simulink model "compare_plant_SIMO"  (R2022b)
settings: Solver=VariableStepAuto  StartTime=0.0  StopTime=100  RelTol=1e-3
values from neighbouring files (symbols this model uses):
  airspeed_trim = 13.8507137299    [airspeed_trim.mat]
  alt_trim = 556.973205566    [alt_trim.mat]
  elevator_trim = 0    [elevator_trim.mat]
  throttle_trim = 0.234714001417    [throttle_trim.mat]
undefined symbols (not defined in the file or in its folder): sigbuilder_block
libraries: simulink_extras x3, dspsrcs4 x1, cstblocks x1

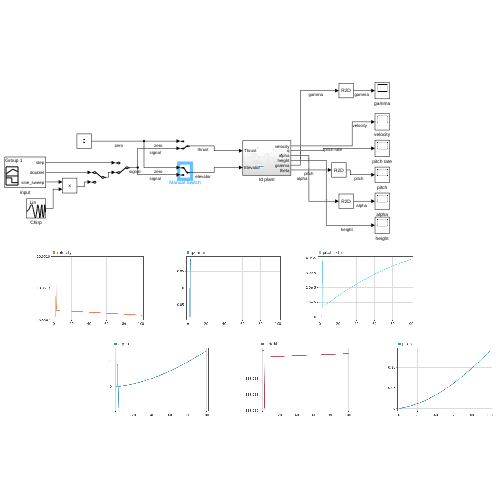
[thumbnail: Simulink's stored preview of the top-level diagram]
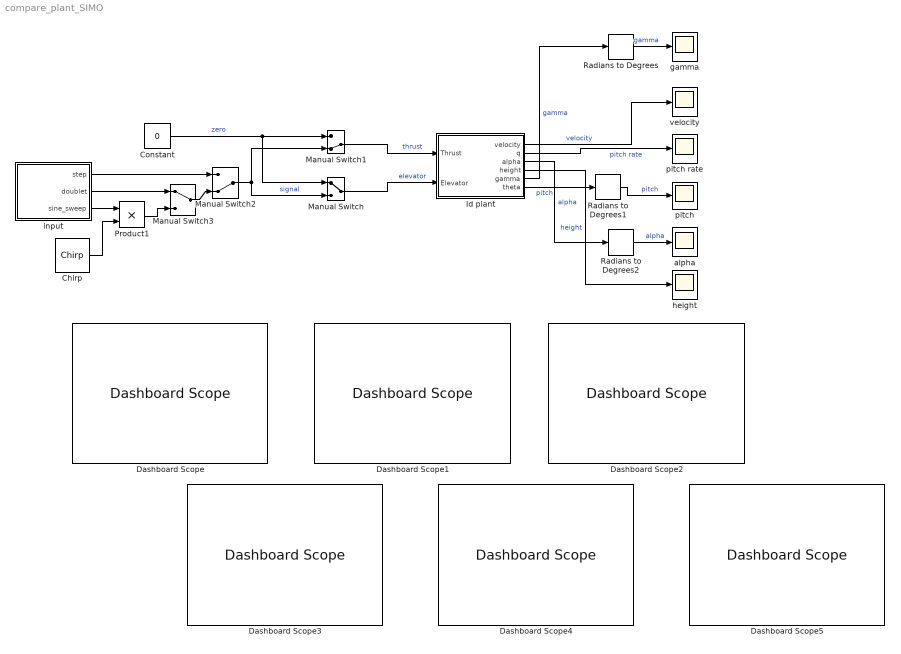
== system compare_plant_SIMO ==
  Chirp : dspsrcs4/Chirp  sweep=Linear  mode=Unidirectional  f0=0  f1=5  t1=20  Tsweep=20  phase=0  Ts=0.02  spf=1  datatype=Double  OutputFrames=off
  Constant : Constant  Value=0
  Dashboard Scope{,1..5} (6 alike) : DashboardScope
  Id plant : Subsystem
  Manual Switch : ManualSwitch
  Manual Switch1 : ManualSwitch  CurrentSetting=0
  Manual Switch2 : ManualSwitch  CurrentSetting=0
  Manual Switch3 : ManualSwitch
  Product1 : Product
  Radians to Degrees : simulink_extras/Transformations/Radians to Degrees
  Radians to Degrees1 : simulink_extras/Transformations/Radians to Degrees
  Radians to Degrees2 : simulink_extras/Transformations/Radians to Degrees
  alpha : Scope
  gamma : Scope
  height : Scope
  input : Subsystem  Tag=STV Subsys  LoadFcn=sigbuilder_block('load');  StartFcn=sigbuilder_block('start');  StopFcn=sigbuilder_block('stop');  ClipboardFcn=sigbuilder_block('clipboard');  mask(Sigbuilder block){tuvar=[0:10]}
      mask help: Simulink:masks:SigbuilderBlock_MD
      mask init:
      | if ~strcmp(get_param(bdroot(gcbh),'SimulationStatus'),'stopped') tuvar = sigbuilder_block('maskInit'); end
  pitch : Scope
  pitch rate : Scope
  velocity : Scope
  wires:
  Manual Switch1/1 -> Id plant/1(Thrust)  "thrust"
  Manual Switch/1 -> Id plant/2("Elevator ")  "elevator"
  Id plant/1(velocity) -> velocity/1  "velocity"
  Id plant/5(gamma) -> Radians to Degrees/1  "gamma"
  Id plant/2(q) -> pitch rate/1  "pitch rate"
  Id plant/3(alpha) -> Radians to Degrees2/1  "alpha"
  Id plant/4(height) -> height/1  "height"
  Product1/1 -> Manual Switch3/2
  Manual Switch2/1 -> Manual Switch/2, Manual Switch1/2  "signal"
  input/1(step) -> Manual Switch2/1
  Constant/1 -> Manual Switch/1, Manual Switch1/1  "zero"
  input/3(sine_sweep) -> Product1/1
  Chirp/1 -> Product1/2
  Id plant/6(theta) -> Radians to Degrees1/1  "pitch"
  Manual Switch3/1 -> Manual Switch2/2
  input/2(doublet) -> Manual Switch3/1
  Radians to Degrees/1 -> gamma/1  "gamma"
  Radians to Degrees1/1 -> pitch/1  "pitch"
  Radians to Degrees2/1 -> alpha/1  "alpha"

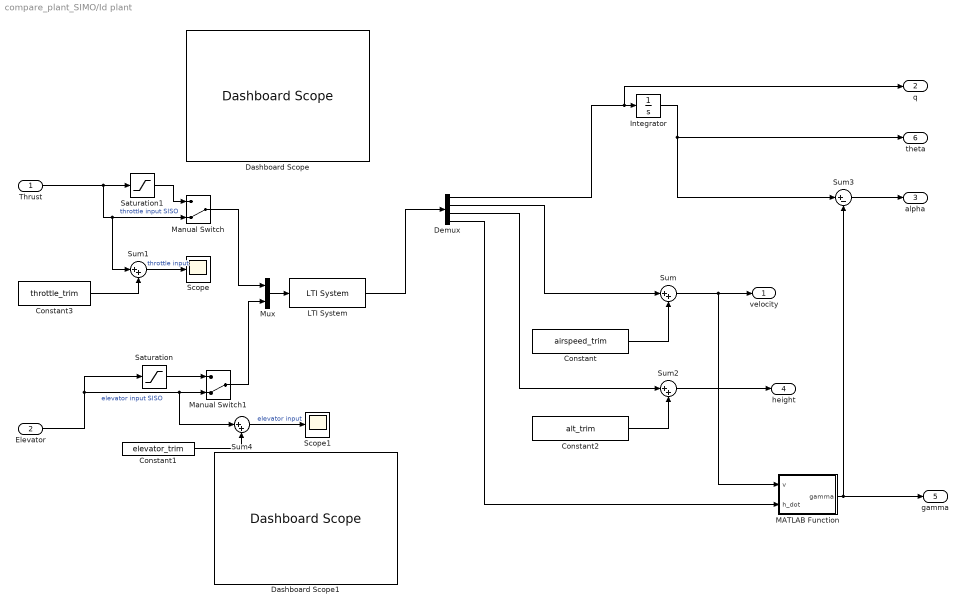
== system compare_plant_SIMO/Id plant ==
  Thrust : Inport
  "Elevator " : Inport  Port=2
  Constant : Constant  Value=airspeed_trim
  Constant1 : Constant  Value=elevator_trim
  Constant2 : Constant  Value=alt_trim
  Constant3 : Constant  Value=throttle_trim
  Dashboard Scope : DashboardScope
  Dashboard Scope1 : DashboardScope
  Demux : Demux
  Integrator : Integrator
  LTI System : cstblocks/LTI System  sys=G2_sitl  IC=[]
  MATLAB Function : MATLAB Function  TreatAsAtomicUnit=on
  Manual Switch : ManualSwitch  CurrentSetting=0
  Manual Switch1 : ManualSwitch  CurrentSetting=0
  Mux : Mux  Inputs=2
  Saturation : Saturate  UpperLimit=deg2rad(30)  LowerLimit=-deg2rad(30)
  Saturation1 : Saturate  UpperLimit=1  LowerLimit=0
  Scope : Scope
  Scope1 : Scope
  Sum{,1..2,4} (4 alike) : Sum  Inputs=|++
  Sum3 : Sum  Inputs=|+-
  velocity : Outport
  q : Outport  Port=2
  alpha : Outport  Port=3
  height : Outport  Port=4
  gamma : Outport  Port=5
  theta : Outport  Port=6
  wires:
  Thrust/1 -> Sum1/1, Manual Switch/2, Saturation1/1  "throttle input SISO"
  Demux/1 -> q/1, Integrator/1
  "Elevator "/1 -> Saturation/1, Sum4/1, Manual Switch1/2  "elevator input SISO"
  Saturation1/1 -> Manual Switch/1
  Saturation/1 -> Manual Switch1/1
  Constant/1 -> Sum/2
  Sum/1 -> MATLAB Function/1(v), velocity/1
  Sum2/1 -> height/1
  Constant2/1 -> Sum2/2
  Integrator/1 -> Sum3/1, theta/1
  Sum3/1 -> alpha/1
  Demux/2 -> Sum/1
  Demux/3 -> Sum2/1
  Mux/1 -> LTI System/1
  LTI System/1 -> Demux/1
  Manual Switch/1 -> Mux/1
  Manual Switch1/1 -> Mux/2
  Demux/4 -> MATLAB Function/2(h_dot)
  MATLAB Function/1(gamma) -> gamma/1, Sum3/2
  Sum1/1 -> Scope/1  "throttle input"
  Constant3/1 -> Sum1/2
  Constant1/1 -> Sum4/2
  Sum4/1 -> Scope1/1  "elevator input"

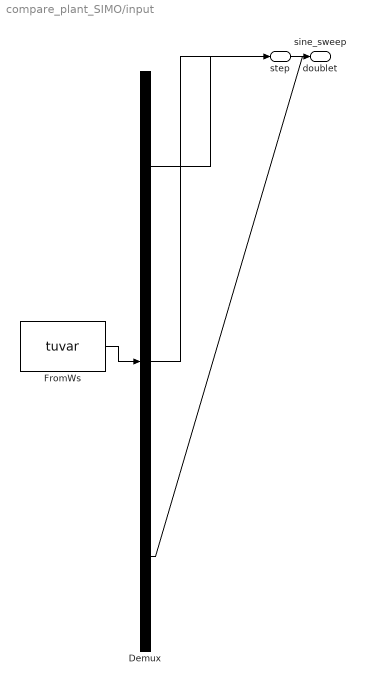
== system compare_plant_SIMO/input ==
  Demux : Demux  Tag=STV Demux  Outputs=3
  FromWs : FromWorkspace  Tag=STV FromWs  VariableName=tuvar  SampleTime=1/50
      SigBuilderData=|
      | common.afterFinalStr = 'Extrapolate'
      | common.sampleTime = '1/50'
      | dataSet.timeRange = [0 20]
      | dataSet.name = 'Group 1'
      | sbobj.Groups.Name = 'Group 1'
      | sbobj.Groups.Signals(1).Name = 'step'
      | sbobj.Groups.Signals(1).XData = [0 1.98 1.98 5.02 20]
      | sbobj.Groups.Signals(1).YData = [0 0 0.1 0.1 0.1]
      | sbobj.Groups.Signals(2).Name = 'doublet'
      | sbobj.Groups.Signals(2).XData = [0 2 2 2.52 2.52 2.98 2.98 20]
      | sbobj.Groups.Signals(2).YData = [0 0 0.1 0.1 -0.1 -0.1 0 0]
      | sbobj.Groups.Signals(3).Name = 'sine_sweep'
      | sbobj.Groups.Signals(3).XData = [0 1.98 1.98 20]
      | sbobj.Groups.Signals(3).YData = [0 0 0.1 0.1]
      | sbobj.Groups.TimeRange = [0 20]
  step : Outport  Tag=STV Outport
  doublet : Outport  Tag=STV Outport  Port=2
  sine_sweep : Outport  Tag=STV Outport  Port=3
  wires:
  Demux/1 -> step/1
  FromWs/1 -> Demux/1
  Demux/2 -> doublet/1
  Demux/3 -> sine_sweep/1

== matlab function compare_plant_SIMO/Id plant/MATLAB Function ==
function gamma = fcn(v,h_dot)

gamma = h_dot/v;
